simulink model "RespiratorySys"  (R2019b)
settings: Solver=VariableStepAuto  StartTime=0.0  StopTime=10.0  RelTol=1e-3
values from neighbouring files (symbols this model uses):
  alpha1 = 0.03198    [xFinalDisease.m]
  alpha2 = 0.05591    [xFinalDisease.m]
  beta1 = 0.008275    [xFinalDisease.m]
  beta2 = 0.03255    [xFinalDisease.m]
  CsatCO2 = 1.9488    [xFinalDisease.m]
  CsatO2 = 0.2128    [xFinalDisease.m]
  CvCO2_IC = 0.522    [xFinalDisease.m]
  CvO2_IC = 0.156    [xFinalDisease.m]
  FICO2 = 0.0/100    (= 0)    [xFinalDisease.m]
  FIO2 = 21.0/100    (= 0.21)    [xFinalDisease.m]
  h1 = 0.3836    [xFinalDisease.m]
  h2 = 1.819    [xFinalDisease.m]
  K1 = 15.0    (= 15)    [xFinalDisease.m]
  K2 = 194.4    [xFinalDisease.m]
  kEff = 1    [xFinalDisease.m]
  PACO2_IC = 40.0    (= 40)    [xFinalDisease.m]
  PAO2_IC = 97.0    (= 97)    [xFinalDisease.m]
  Patm = 760.0    (= 760)    [xFinalDisease.m]
  PdCO2_IC = 38.0    (= 38)    [xFinalDisease.m]
  PdO2_IC = 100.0    (= 100)    [xFinalDisease.m]
  Pws = 47.0    (= 47)    [xFinalDisease.m]
  Rlung = 0.24    [xFinalDisease.m]
  Rtube = 3.76    [xFinalDisease.m]
  shunt = 1.5/100    (= 0.015)    [xFinalDisease.m]
  Tau_TL = 10.0    (= 10)    [xFinalDisease.m]
  Tsamp = 1e-3    (= 0.001)    [xFinalDisease.m]
  VD = 0.125    [xFinalDisease.m]
  VL0 = 3.40    (= 3.4)    [xFinalDisease.m]
  VReference = 0.45    [xFinalDisease.m]
libraries: fl_lib x10, nesl_utility x4, simulink x2
settings Model: Creator=SÜLEYMAN  LastModifiedBy=SÜLEYMAN

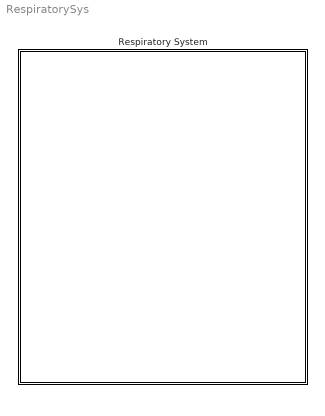
== system RespiratorySys ==
  Respiratory System : Subsystem

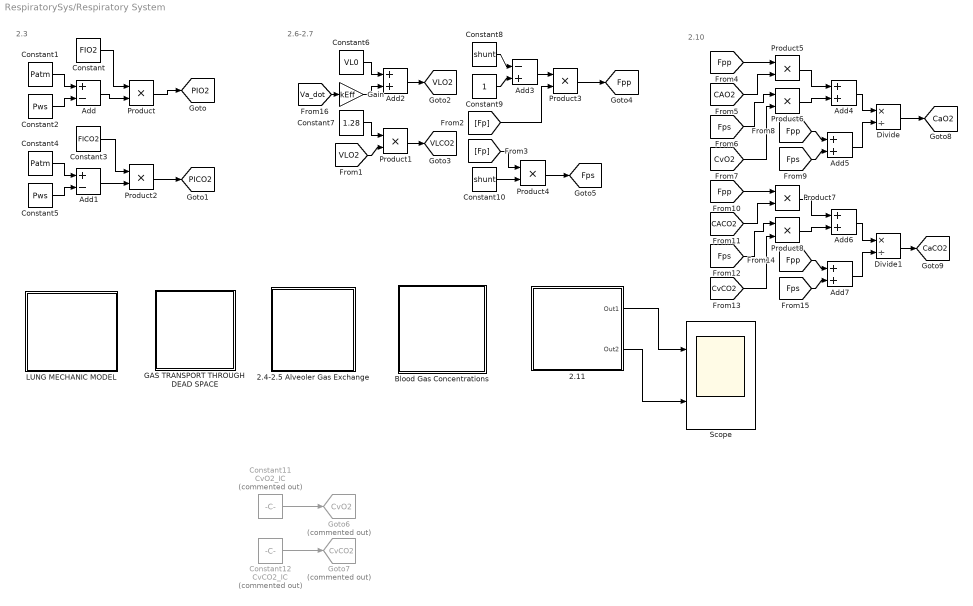
== system RespiratorySys/Respiratory System ==
  note: 2.10
  note: 2.6-2.7
  note: 2.3
  "2.11 " : Subsystem
  2.4-2.5 Alveoler Gas Exchange : Subsystem
  Add : Sum  Inputs=+-
  Add1 : Sum  Inputs=+-
  Add{2,4..7} (5 alike) : Sum
  Add3 : Sum  Inputs=-+
  "Blood Gas Concentrations " : Subsystem
  Constant : Constant  Value=FIO2  SampleTime=Tsamp
  Constant1 : Constant  Value=Patm  SampleTime=Tsamp
  Constant10 : Constant  Value=shunt  SampleTime=Tsamp
  Constant11 : Constant  Commented=on  Value=CvO2_IC  SampleTime=Tsamp
  Constant12 : Constant  Commented=on  Value=CvCO2_IC  SampleTime=Tsamp
  Constant2 : Constant  Value=Pws  SampleTime=Tsamp
  Constant3 : Constant  Value=FICO2  SampleTime=Tsamp
  Constant4 : Constant  Value=Patm  SampleTime=Tsamp
  Constant5 : Constant  Value=Pws  SampleTime=Tsamp
  Constant6 : Constant  Value=VL0  SampleTime=Tsamp
  Constant7 : Constant  Value=1.28  SampleTime=Tsamp
  Constant8 : Constant  Value=shunt  SampleTime=Tsamp
  Constant9 : Constant  SampleTime=Tsamp
  Divide : Product  Inputs=*/
  Divide1 : Product  Inputs=*/
  GAS TRANSPORT THROUGH DEAD SPACE : Subsystem
  Gain : Gain  Gain=kEff
  Goto6 : Goto  Commented=on  GotoTag=CvO2  TagVisibility=global
  Goto7 : Goto  Commented=on  GotoTag=CvCO2  TagVisibility=global
  LUNG MECHANIC MODEL : Subsystem
  Product{,1..8} (9 alike) : Product
  Scope : Scope  NumInputPorts=2
  tag scope: CaCO2=global, CaO2=global, Fpp=global, Fps=global, PICO2=global, PIO2=global, VLCO2=global, VLO2=global
  wires:
  Constant9/1 -> Add3/2
  Add5/1 -> Divide/2
  Constant2/1 -> Add/2
  Constant10/1 -> Product4/2
  Constant8/1 -> Add3/1
  Add4/1 -> Divide/1
  [Fp] -> Product3/2
  Add2/1 -> [VLO2]
  [CvO2] -> Product6/2
  Constant5/1 -> Add1/2
  Constant7/1 -> Product1/1
  [VLO2] -> Product1/2
  Constant3/1 -> Product2/1
  [Fp] -> Product4/1
  Add3/1 -> Product3/1
  Constant1/1 -> Add/1
  Product5/1 -> Add4/1
  Product8/1 -> Add6/2
  Constant4/1 -> Add1/1
  Product3/1 -> [Fpp]
  Gain/1 -> Add2/2
  [Fps] -> Add7/2
  Product1/1 -> [VLCO2]
  [Fpp] -> Add7/1
  Product2/1 -> [PICO2]
  Add/1 -> Product/2
  Add1/1 -> Product2/2
  Constant6/1 -> Add2/1
  Add6/1 -> Divide1/1
  [CvCO2] -> Product8/2
  [CACO2] -> Product7/2
  Product6/1 -> Add4/2
  [CAO2] -> Product5/2
  Product4/1 -> [Fps]
  [Fpp] -> Add5/1
  Constant/1 -> Product/1
  Product7/1 -> Add6/1
  Divide1/1 -> [CaCO2]
  Product/1 -> [PIO2]
  [Va_dot] -> Gain/1
  [Fps] -> Product8/1
  [Fpp] -> Product5/1
  [Fps] -> Add5/2
  Add7/1 -> Divide1/2
  [Fps] -> Product6/1
  [Fpp] -> Product7/1
  Divide/1 -> [CaO2]
  Constant11/1 -> Goto6/1
  Constant12/1 -> Goto7/1
  "2.11 "/1(Out1) -> Scope/1
  "2.11 "/2(Out2) -> Scope/2

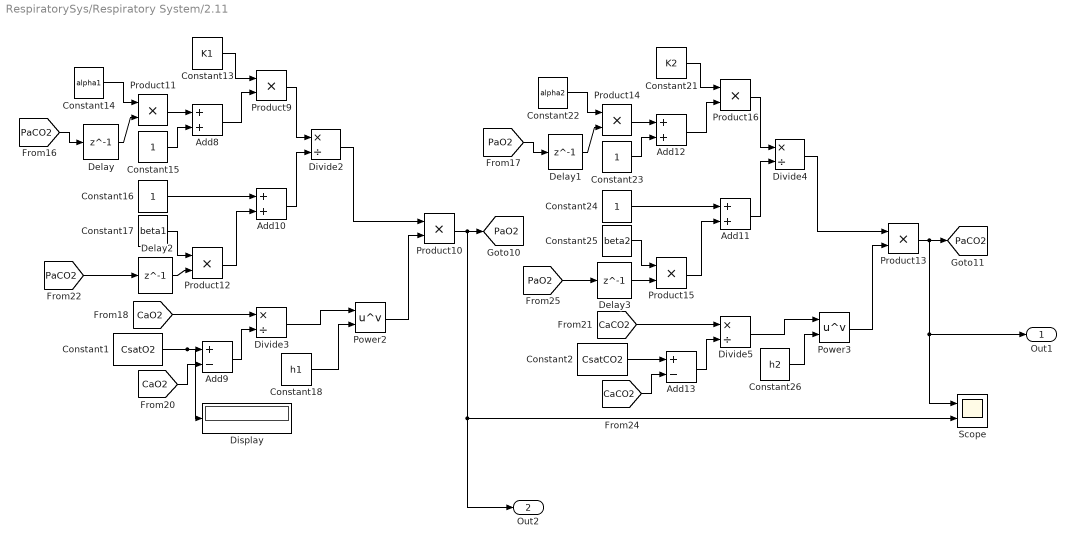
== system RespiratorySys/Respiratory System/2.11  ==
  Add{8,10..12} (4 alike) : Sum
  Add13 : Sum  Inputs=+-
  Add9 : Sum  Inputs=+-
  Constant1 : Constant  Value=CsatO2  SampleTime=Tsamp
  Constant13 : Constant  Value=K1  SampleTime=Tsamp
  Constant14 : Constant  Value=alpha1  SampleTime=Tsamp
  Constant{15..16,23..24} (4 alike) : Constant  SampleTime=Tsamp
  Constant17 : Constant  Value=beta1  SampleTime=Tsamp
  Constant18 : Constant  Value=h1  SampleTime=Tsamp
  Constant2 : Constant  Value=CsatCO2  SampleTime=Tsamp
  Constant21 : Constant  Value=K2  SampleTime=Tsamp
  Constant22 : Constant  Value=alpha2  SampleTime=Tsamp
  Constant25 : Constant  Value=beta2  SampleTime=Tsamp
  Constant26 : Constant  Value=h2  SampleTime=Tsamp
  Delay : Delay  DelayLength=1  SampleTime=Tsamp
  Delay1 : Delay  DelayLength=1  InitialCondition=0  SampleTime=Tsamp
  Delay2 : Delay  DelayLength=1  InitialCondition=0  SampleTime=Tsamp
  Delay3 : Delay  DelayLength=1  InitialCondition=0  SampleTime=Tsamp
  Display : Display
  Divide{2..5} (4 alike) : Product  Inputs=*/
  Power2 : Math  Operator=pow  SignedPower=off  SaturateOnIntegerOverflow=on
  Power3 : Math  Operator=pow  SignedPower=off  SaturateOnIntegerOverflow=on
  Product{9..16} (8 alike) : Product
  Scope : Scope  NumInputPorts=2
  Out1 : Outport
  Out2 : Outport  Port=2
  tag scope: PaCO2=global, PaO2=global
  wires:
  Constant2/1 -> Add13/1
  Constant22/1 -> Product14/1
  [CaO2] -> Divide3/1
  Divide4/1 -> Product13/1
  Constant21/1 -> Product16/1
  Constant15/1 -> Add8/2
  Add12/1 -> Product16/2
  Add10/1 -> Divide2/2
  Product13/1 -> Out1/1, Scope/1, [PaCO2]
  Constant1/1 -> Display/1, Add9/1
  Add13/1 -> Divide5/2
  Product15/1 -> Add11/2
  Constant25/1 -> Product15/1
  [PaCO2] -> Delay/1
  Constant24/1 -> Add11/1
  Delay/1 -> Product11/2
  Delay1/1 -> Product14/2
  Product11/1 -> Add8/1
  [PaO2] -> Delay1/1
  Product10/1 -> Out2/1, Scope/2, [PaO2]
  [CaCO2] -> Add13/2
  Product12/1 -> Add10/2
  Product16/1 -> Divide4/1
  Constant14/1 -> Product11/1
  Power3/1 -> Product13/2
  Constant23/1 -> Add12/2
  [CaCO2] -> Divide5/1
  Add11/1 -> Divide4/2
  Product14/1 -> Add12/1
  Constant17/1 -> Product12/1
  Constant16/1 -> Add10/1
  Constant13/1 -> Product9/1
  Product9/1 -> Divide2/1
  Power2/1 -> Product10/2
  Add8/1 -> Product9/2
  [CaO2] -> Add9/2
  Divide2/1 -> Product10/1
  Add9/1 -> Divide3/2
  [PaCO2] -> Delay2/1
  Delay2/1 -> Product12/2
  Divide3/1 -> Power2/1
  Constant18/1 -> Power2/2
  Divide5/1 -> Power3/1
  Constant26/1 -> Power3/2
  [PaO2] -> Delay3/1
  Delay3/1 -> Product15/2

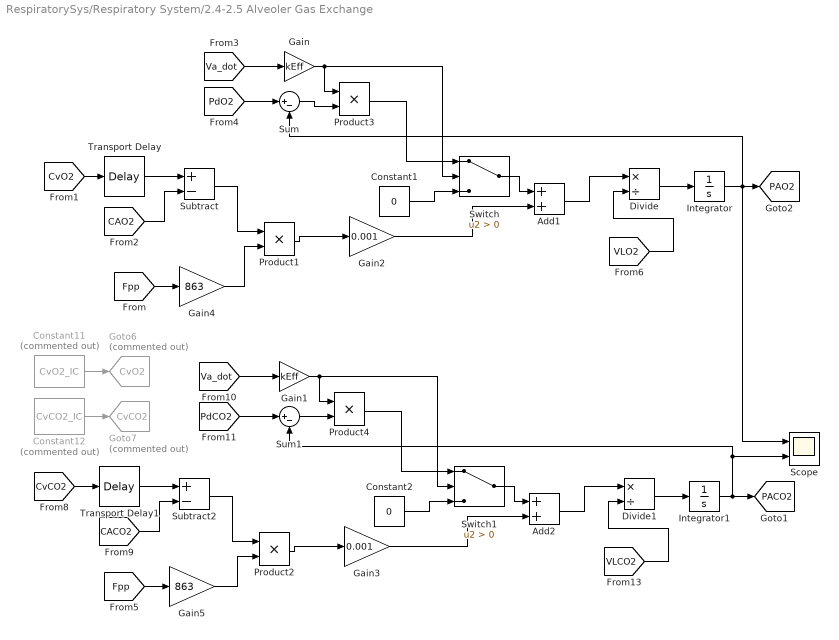
== system RespiratorySys/Respiratory System/2.4-2.5 Alveoler Gas Exchange ==
  Add1 : Sum
  Add2 : Sum
  Constant1 : Constant  Value=0  SampleTime=Tsamp
  Constant11 : Constant  Commented=on  Value=CvO2_IC  SampleTime=Tsamp
  Constant12 : Constant  Commented=on  Value=CvCO2_IC  SampleTime=Tsamp
  Constant2 : Constant  Value=0  SampleTime=Tsamp
  Divide : Product  Inputs=*/
  Divide1 : Product  Inputs=*/
  Gain : Gain  Gain=kEff
  Gain1 : Gain  Gain=kEff
  Gain2 : Gain  Gain=0.001
  Gain3 : Gain  Gain=0.001
  Gain4 : Gain  Gain=863
  Gain5 : Gain  Gain=863
  Goto6 : Goto  Commented=on  GotoTag=CvO2  TagVisibility=global
  Goto7 : Goto  Commented=on  GotoTag=CvCO2  TagVisibility=global
  Integrator : Integrator  InitialCondition=PAO2_IC
  Integrator1 : Integrator  InitialCondition=PACO2_IC
  Product{1..4} (4 alike) : Product
  Scope : Scope  NumInputPorts=2
  Subtract : Sum  Inputs=+-
  Subtract2 : Sum  Inputs=+-
  Sum : Sum  Inputs=|+-
  Sum1 : Sum  Inputs=|+-
  Switch : Switch  Criteria=u2 > Threshold
  Switch1 : Switch  Criteria=u2 > Threshold
  Transport Delay : TransportDelay  DelayTime=Tau_TL  InitialOutput=CvO2_IC  BufferSize=10240  FixedBuffer=on
  Transport Delay1 : TransportDelay  DelayTime=Tau_TL  InitialOutput=CvCO2_IC  BufferSize=10240  FixedBuffer=on
  tag scope: PACO2=global, PAO2=global
  wires:
  Product3/1 -> Switch/1
  Subtract/1 -> Product1/1
  [CAO2] -> Subtract/2
  [Va_dot] -> Gain/1
  Gain/1 -> Product3/1, Switch/2
  Transport Delay/1 -> Subtract/1
  [CvO2] -> Transport Delay/1
  Divide/1 -> Integrator/1
  [PdO2] -> Sum/1
  Integrator/1 -> Sum/2, Scope/1, [PAO2]
  Sum/1 -> Product3/2
  [VLO2] -> Divide/2
  Product1/1 -> Gain2/1
  Constant1/1 -> Switch/3
  Switch/1 -> Add1/1
  Gain2/1 -> Add1/2
  Add1/1 -> Divide/1
  [PdCO2] -> Sum1/1
  [CvCO2] -> Transport Delay1/1
  Subtract2/1 -> Product2/1
  [CACO2] -> Subtract2/2
  Divide1/1 -> Integrator1/1
  Switch1/1 -> Add2/1
  Integrator1/1 -> Sum1/2, Scope/2, [PACO2]
  Transport Delay1/1 -> Subtract2/1
  Sum1/1 -> Product4/2
  Product4/1 -> Switch1/1
  Constant2/1 -> Switch1/3
  [VLCO2] -> Divide1/2
  Product2/1 -> Gain3/1
  Add2/1 -> Divide1/1
  [Va_dot] -> Gain1/1
  Gain3/1 -> Add2/2
  Gain1/1 -> Product4/1, Switch1/2
  [Fpp] -> Gain4/1
  Gain4/1 -> Product1/2
  Gain5/1 -> Product2/2
  [Fpp] -> Gain5/1
  Constant12/1 -> Goto7/1
  Constant11/1 -> Goto6/1

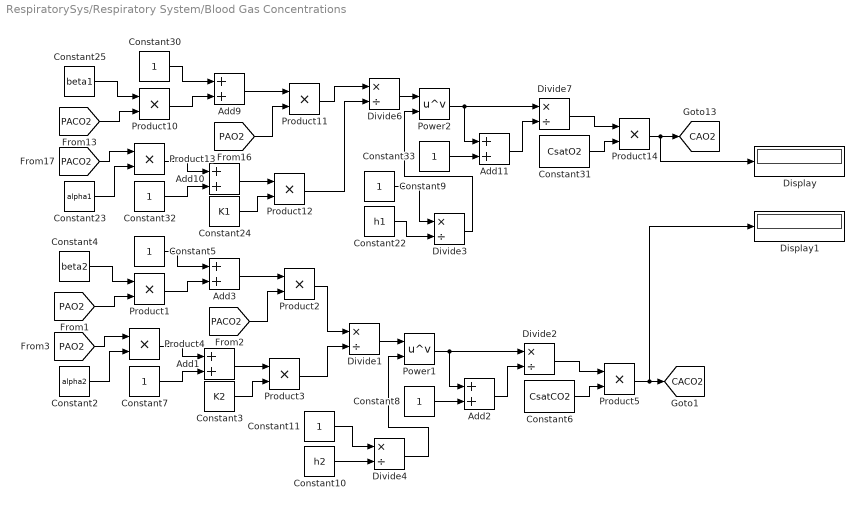
== system RespiratorySys/Respiratory System/Blood Gas Concentrations  ==
  Add{1..3,9..11} (6 alike) : Sum
  Constant10 : Constant  Value=h2  SampleTime=Tsamp
  Constant{5,7..9,11,30,32..33} (8 alike) : Constant  SampleTime=Tsamp
  Constant2 : Constant  Value=alpha2  SampleTime=Tsamp
  Constant22 : Constant  Value=h1  SampleTime=Tsamp
  Constant23 : Constant  Value=alpha1  SampleTime=Tsamp
  Constant24 : Constant  Value=K1  SampleTime=Tsamp
  Constant25 : Constant  Value=beta1  SampleTime=Tsamp
  Constant3 : Constant  Value=K2  SampleTime=Tsamp
  Constant31 : Constant  Value=CsatO2  SampleTime=Tsamp
  Constant4 : Constant  Value=beta2  SampleTime=Tsamp
  Constant6 : Constant  Value=CsatCO2  SampleTime=Tsamp
  Display : Display
  Display1 : Display
  Divide{1..4,6..7} (6 alike) : Product  Inputs=*/
  Power1 : Math  Operator=pow  SignedPower=off  SaturateOnIntegerOverflow=on
  Power2 : Math  Operator=pow  SignedPower=off  SaturateOnIntegerOverflow=on
  Product{1..5,10..14} (10 alike) : Product
  tag scope: CACO2=global, CAO2=global
  wires:
  Constant24/1 -> Product12/2
  Power2/1 -> Add11/1, Divide7/1
  Add10/1 -> Product12/1
  Product10/1 -> Add9/2
  Divide7/1 -> Product14/1
  Product12/1 -> Divide6/2
  Product13/1 -> Add10/1
  Constant33/1 -> Add11/2
  Constant23/1 -> Product13/2
  Constant30/1 -> Add9/1
  Add9/1 -> Product11/1
  Constant32/1 -> Add10/2
  Product14/1 -> Display/1, [CAO2]
  Constant25/1 -> Product10/1
  [PAO2] -> Product11/2
  Add11/1 -> Divide7/2
  Product11/1 -> Divide6/1
  Constant31/1 -> Product14/2
  [PACO2] -> Product10/2
  [PACO2] -> Product13/1
  Add3/1 -> Product2/1
  Constant2/1 -> Product4/2
  Constant5/1 -> Add3/1
  Constant8/1 -> Add2/2
  Divide2/1 -> Product5/1
  Add1/1 -> Product3/1
  Power1/1 -> Add2/1, Divide2/1
  Product1/1 -> Add3/2
  Product3/1 -> Divide1/2
  Constant3/1 -> Product3/2
  Product4/1 -> Add1/1
  Add2/1 -> Divide2/2
  Product5/1 -> Display1/1, [CACO2]
  Product2/1 -> Divide1/1
  [PAO2] -> Product4/1
  Constant7/1 -> Add1/2
  [PACO2] -> Product2/2
  Constant4/1 -> Product1/1
  [PAO2] -> Product1/2
  Constant6/1 -> Product5/2
  Divide1/1 -> Power1/1
  Divide4/1 -> Power1/2
  Divide6/1 -> Power2/1
  Constant22/1 -> Divide3/2
  Divide3/1 -> Power2/2
  Constant9/1 -> Divide3/1
  Constant11/1 -> Divide4/1
  Constant10/1 -> Divide4/2

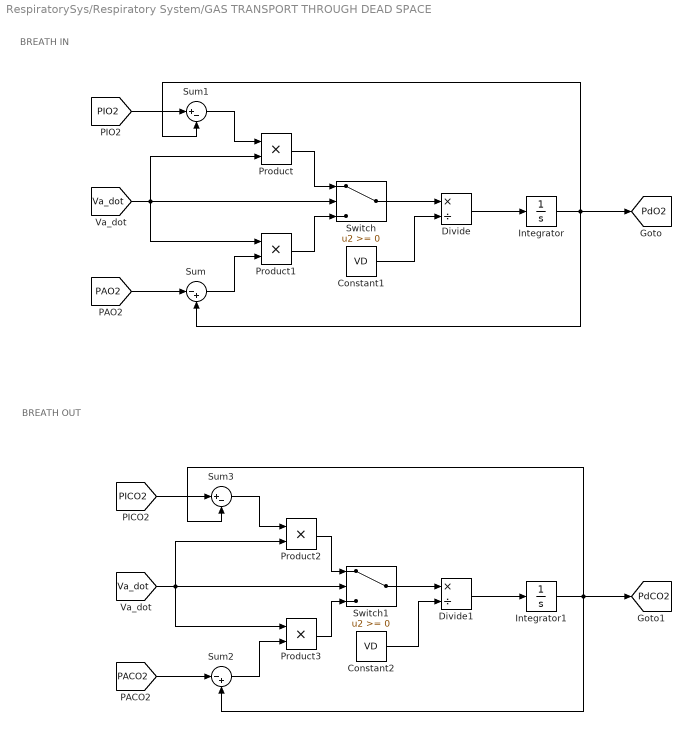
== system RespiratorySys/Respiratory System/GAS TRANSPORT THROUGH DEAD SPACE ==
  note: BREATH IN
  note: BREATH OUT
  Constant1 : Constant  Value=VD  SampleTime=Tsamp
  Constant2 : Constant  Value=VD  SampleTime=Tsamp
  Divide : Product  Inputs=*/
  Divide1 : Product  Inputs=*/
  Integrator : Integrator  InitialCondition=PdO2_IC
  Integrator1 : Integrator  InitialCondition=PdCO2_IC
  Product{,1..3} (4 alike) : Product
  Sum : Sum  Inputs=|-+
  Sum1 : Sum  Inputs=|+-
  Sum2 : Sum  Inputs=|-+
  Sum3 : Sum  Inputs=|+-
  Switch : Switch
  Switch1 : Switch
  tag scope: PdCO2=global, PdO2=global
  wires:
  Integrator1/1 -> [PdCO2], Sum2/2, Sum3/2
  Product1/1 -> Switch/3
  [Va_dot] -> Switch/2, Product1/1, Product/2
  [PIO2] -> Sum1/1
  Integrator/1 -> [PdO2], Sum/2, Sum1/2
  Sum1/1 -> Product/1
  Sum/1 -> Product1/2
  Switch/1 -> Divide/1
  [Va_dot] -> Switch1/2, Product3/1, Product2/2
  [PICO2] -> Sum3/1
  Product/1 -> Switch/1
  Constant1/1 -> Divide/2
  Divide1/1 -> Integrator1/1
  Constant2/1 -> Divide1/2
  Product2/1 -> Switch1/1
  Divide/1 -> Integrator/1
  [PACO2] -> Sum2/1
  Sum2/1 -> Product3/2
  Switch1/1 -> Divide1/1
  Product3/1 -> Switch1/3
  Sum3/1 -> Product2/1
  [PAO2] -> Sum/1

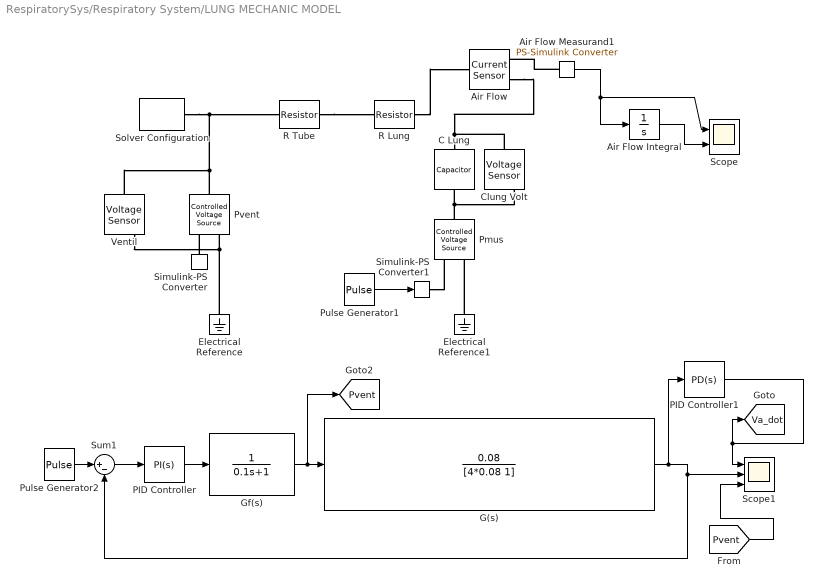
== system RespiratorySys/Respiratory System/LUNG MECHANIC MODEL ==
  Air Flow : fl_lib/Electrical/Electrical Sensors/Current Sensor
  Air Flow Measurand1 : nesl_utility/PS-Simulink Converter  PhysicalDomain=network_engine_domain  SubClassName=ps_output  LeftPortType=input  RightPortType=output  PseudoPeriodic=off  Frequencies=[]  Unit=inherit  AffineConversion=off
  Air Flow Integral : Integrator  InitialCondition=VReference
  C Lung : fl_lib/Electrical/Electrical Elements/Capacitor  c=Clung F  r=Clung Ohm  g=0 1/Ohm  i_specify=off  i_priority=None  i=0 A  i_nominal_specify=off  i_nominal_unit=A  i_nominal_value=1  v_specify=off  v_priority=None  v=0 V  v_nominal_specify=off  v_nominal_unit=V  v_nominal_value=1  vc_specify=off  vc_priority=High  vc=0 V  vc_nominal_specify=off  vc_nominal_unit=V  vc_nominal_value=1
  Clung Volt : fl_lib/Electrical/Electrical Sensors/Voltage Sensor
  Electrical Reference : fl_lib/Electrical/Electrical Elements/Electrical Reference
  Electrical Reference1 : fl_lib/Electrical/Electrical Elements/Electrical Reference
  "G(s) " : TransferFcn  Numerator=[0.08]  Denominator=[4*0.08 1]
  "Gf(s) " : TransferFcn  Denominator=[0.1 1]
  PID Controller : simulink/Continuous/PID Controller  Controller=PI  Form=Parallel  TimeDomain=Continuous-time  SampleTime=-1  IntegratorMethod=Forward Euler  FilterMethod=Forward Euler  ControllerParametersSource=internal  P=11.56  I=3.125*11.56  D=0  UseFilter=on  N=100  TunerSelectOption=Transfer Function Based (PID Tuner App)  InitialConditionSource=internal  InitialConditionForIntegrator=0  InitialConditionForFilter=0  DifferentiatorICPrevScaledInput=0  ExternalReset=none  TrackingMode=off  Kt=1  LimitOutput=on  UpperSaturationLimit=inf  LowerSaturationLimit=0  LinearizeAsGain=on  AntiWindupMode=back-calculation  Kb=1  POutMin=[]  POutMax=[]  IOutMin=[]  IOutMax=[]  DOutMin=[]  DOutMax=[]  NOutMin=[]  NOutMax=[]  SumOutMin=[]  SumOutMax=[]  SaturationOutMin=[]  SaturationOutMax=[]  PParamMin=[]  PParamMax=[]  IParamMin=[]  IParamMax=[]  DParamMin=[]  DParamMax=[]  NParamMin=[]  NParamMax=[]  KbParamMin=[]  KbParamMax=[]  KtParamMin=[]  KtParamMax=[]  KbOutMin=[]  KbOutMax=[]  KtOutMin=[]  KtOutMax=[]  IntegratorOutMin=[]  IntegratorOutMax=[]  FilterOutMin=[]  FilterOutMax=[]  SumI1OutMin=[]  SumI1OutMax=[]  SumI2OutMin=[]  SumI2OutMax=[]  SumI3OutMin=[]  SumI3OutMax=[]  SumI4OutMin=[]  SumI4OutMax=[]  SumDOutMin=[]  SumDOutMax=[]  DifferentiatorOutMin=[]  DifferentiatorOutMax=[]  FilterDiffOutCoefMin=[]  FilterDiffOutCoefMax=[]  ReciprocalOutMin=[]  ReciprocalOutMax=[]  SumDenOutMin=[]  SumDenOutMax=[]  SumNumOutMin=[]  SumNumOutMax=[]  DivideOutMin=[]  DivideOutMax=[]  IntegratorContinuousStateAttributes=''  IntegratorStateMustResolveToSignalObject=off  IntegratorRTWStateStorageClass=Auto  FilterContinuousStateAttributes=''  FilterStateMustResolveToSignalObject=off  FilterRTWStateStorageClass=Auto  ParallelPVariant=InternalParameters  IdealPVariant=Disabled  IVariant=InternalParameters  DVariant=Disabled  IntegratorVariant=Continuous  SatVariant=Enabled  AWVariant=BackCalculation  PCopyVariant=Disabled  TRVariant=Disabled  FdbkBlocksVariant=Forward  IdealPFdbkVariant=Disabled  SatFdbkVariant=Disabled  DerivativeFilterVariant=Disabled  NVariant=Disabled  NCopyVariant=Disabled_SignalSpec  FilterICVariant=Disabled  IntegratorICVariant=InternalICs  ExternalResetVariant=Disabled  TRSumVariant=Passthrough  SumFdbkVariant=Disabled  SumVariant=Sum_PI
  PID Controller1 : simulink/Continuous/PID Controller  Controller=PD  Form=Parallel  TimeDomain=Continuous-time  SampleTime=-1  IntegratorMethod=Forward Euler  FilterMethod=Forward Euler  ControllerParametersSource=internal  P=0  I=36.125  D=1  UseFilter=on  N=100  TunerSelectOption=Transfer Function Based (PID Tuner App)  InitialConditionSource=internal  InitialConditionForIntegrator=0  InitialConditionForFilter=0  DifferentiatorICPrevScaledInput=0  ExternalReset=none  TrackingMode=off  Kt=1  LimitOutput=on  UpperSaturationLimit=inf  LowerSaturationLimit=-inf  LinearizeAsGain=on  AntiWindupMode=back-calculation  Kb=1  POutMin=[]  POutMax=[]  IOutMin=[]  IOutMax=[]  DOutMin=[]  DOutMax=[]  NOutMin=[]  NOutMax=[]  SumOutMin=[]  SumOutMax=[]  SaturationOutMin=[]  SaturationOutMax=[]  PParamMin=[]  PParamMax=[]  IParamMin=[]  IParamMax=[]  DParamMin=[]  DParamMax=[]  NParamMin=[]  NParamMax=[]  KbParamMin=[]  KbParamMax=[]  KtParamMin=[]  KtParamMax=[]  KbOutMin=[]  KbOutMax=[]  KtOutMin=[]  KtOutMax=[]  IntegratorOutMin=[]  IntegratorOutMax=[]  FilterOutMin=[]  FilterOutMax=[]  SumI1OutMin=[]  SumI1OutMax=[]  SumI2OutMin=[]  SumI2OutMax=[]  SumI3OutMin=[]  SumI3OutMax=[]  SumI4OutMin=[]  SumI4OutMax=[]  SumDOutMin=[]  SumDOutMax=[]  DifferentiatorOutMin=[]  DifferentiatorOutMax=[]  FilterDiffOutCoefMin=[]  FilterDiffOutCoefMax=[]  ReciprocalOutMin=[]  ReciprocalOutMax=[]  SumDenOutMin=[]  SumDenOutMax=[]  SumNumOutMin=[]  SumNumOutMax=[]  DivideOutMin=[]  DivideOutMax=[]  IntegratorContinuousStateAttributes=''  IntegratorStateMustResolveToSignalObject=off  IntegratorRTWStateStorageClass=Auto  FilterContinuousStateAttributes=''  FilterStateMustResolveToSignalObject=off  FilterRTWStateStorageClass=Auto  ParallelPVariant=InternalParameters  IdealPVariant=Disabled  IVariant=Disabled  DVariant=InternalParameters  IntegratorVariant=Disabled  SatVariant=Enabled  AWVariant=Disabled  PCopyVariant=Disabled  TRVariant=Disabled  FdbkBlocksVariant=Forward  IdealPFdbkVariant=Disabled  SatFdbkVariant=Disabled  DerivativeFilterVariant=ContFilter  NVariant=InternalParameters  NCopyVariant=Disabled  FilterICVariant=InternalICsFilter  IntegratorICVariant=Disabled  ExternalResetVariant=Disabled  TRSumVariant=Passthrough  SumFdbkVariant=Disabled  SumVariant=Sum_PD
  Pmus : fl_lib/Electrical/Electrical Sources/Controlled Voltage Source
  Pulse Generator1 : DiscretePulseGenerator  PulseType=Time based  Amplitude=0  Period=5  PulseWidth=35
  Pulse Generator2 : DiscretePulseGenerator  PulseType=Time based  Amplitude=VReference  Period=5  PulseWidth=35
  Pvent : fl_lib/Electrical/Electrical Sources/Controlled Voltage Source
  R Lung : fl_lib/Electrical/Electrical Elements/Resistor  R=Rlung Ohm  i_specify=off  i_priority=None  i=0 A  i_nominal_specify=off  i_nominal_unit=A  i_nominal_value=1  v_specify=off  v_priority=None  v=0 V  v_nominal_specify=off  v_nominal_unit=V  v_nominal_value=1
  R Tube : fl_lib/Electrical/Electrical Elements/Resistor  R=Rtube Ohm  i_specify=off  i_priority=None  i=0 A  i_nominal_specify=off  i_nominal_unit=A  i_nominal_value=1  v_specify=off  v_priority=None  v=0 V  v_nominal_specify=off  v_nominal_unit=V  v_nominal_value=1
  Scope : Scope  NumInputPorts=2
  Scope1 : Scope  NumInputPorts=3
  Simulink-PS Converter : nesl_utility/Simulink-PS Converter  PhysicalDomain=network_engine_domain  SubClassName=ps_input  LeftPortType=input  RightPortType=output  PseudoPeriodic=off  Frequencies=[]  NoiseDistribution=none  NoiseParameters=[]  Unit=1  AffineConversion=off  FilteringAndDerivatives=provide  SimscapeFilterOrder=1  InputFilterTimeConstant=0.001  UdotUserProvided=0
  Simulink-PS Converter1 : nesl_utility/Simulink-PS Converter  PhysicalDomain=network_engine_domain  SubClassName=ps_input  LeftPortType=input  RightPortType=output  PseudoPeriodic=off  Frequencies=[]  NoiseDistribution=none  NoiseParameters=[]  Unit=1  AffineConversion=off  FilteringAndDerivatives=provide  SimscapeFilterOrder=1  InputFilterTimeConstant=0.001  UdotUserProvided=0
  Solver Configuration : nesl_utility/Solver Configuration  PhysicalDomain=network_engine_domain  SubClassName=solver  LeftPortType=input  RightPortType=generic  Tones=[]  Harmonics=[]  SimulateNoise=off  Profile=off  UseLocalSampling=off  EnableSwitchedLinearOptims=on  FrequencyDomain=off  UseCCode=off  RelTol=0.001  AbsTol=1e-06  MinStep=1e-09  ToWorkspace=off  RevertToSquareIcSolve=off  NumHomotopyIterations=100  PhasorMode=off  PhasorModeNumHarmonics=1  DoDC=off  ResidualTolerance=1e-09  UseLocalSolver=off  LocalSolverChoice=NE_BACKWARD_EULER_ADVANCER  LocalSolverSampleTime=0.001  DoFixedCost=off  MaxNonlinIter=3  MaxModeIter=2  LinearAlgebra=auto  EquationFormulation=NE_TIME_EF  DelaysMemoryBudget=1024  AutomaticFiltering=on  FilteringTimeConstant=0.001  PartitionStorageMethod=AS_NEEDED  PartitionMemoryBudget=1024  PartitionMethod=ROBUST
  Sum1 : Sum  Inputs=|+-
  Ventil : fl_lib/Electrical/Electrical Sensors/Voltage Sensor
  tag scope: Pvent=global, Va_dot=global
  wires:
  Pulse Generator1/1 -> Simulink-PS Converter1/1
  Air Flow Measurand1/1 -> Air Flow Integral/1, Scope/1
  Air Flow Integral/1 -> Scope/2
  PID Controller/1 -> "Gf(s) "/1
  Pulse Generator2/1 -> Sum1/1
  Sum1/1 -> PID Controller/1
  "Gf(s) "/1 -> [Pvent], "G(s) "/1
  "G(s) "/1 -> PID Controller1/1, Sum1/2, Scope1/2
  PID Controller1/1 -> [Va_dot], Scope1/1
  [Pvent] -> Scope1/3
  connections:
  R Tube/RConn1 -- R Lung/LConn1
  Air Flow Measurand1/LConn1 -- Air Flow/RConn1
  Clung Volt/LConn1 -- Air Flow/RConn2 -- C Lung/LConn1
  Simulink-PS Converter/RConn1 -- Pvent/RConn1
  R Lung/RConn1 -- Air Flow/LConn1
  Electrical Reference1/LConn1 -- Pmus/RConn2
  Pmus/LConn1 -- Clung Volt/RConn2 -- C Lung/RConn1
  Electrical Reference/LConn1 -- Ventil/RConn2 -- Pvent/RConn2
  Pvent/LConn1 -- Ventil/LConn1 -- Solver Configuration/RConn1 -- R Tube/LConn1
  Simulink-PS Converter1/RConn1 -- Pmus/RConn1
